simulink model "MovementCoord"  (R2016a)
settings: Solver=VariableStepAuto  SolverMode=SingleTasking  StartTime=0.0  StopTime=10.0  RelTol=1e-3
libraries: vrlib x1
settings Model: Creator=HP  LastModifiedBy=kavits
settings DebuggingCC: AlgebraicLoopMsg=none  SFUnexpectedBacktrackingDiag=error  SFNoUnconditionalDefaultTransitionDiag=error
settings GRTTargetCC: TargetLangStandard=C99 (ISO)  GeneratePreprocessorConditionals=Use local settings
settings ConfigComp: CovMetricSettings=dwe  CovHtmlReporting=off  CovSaveCumulativeToWorkspaceVar=off  CovSaveSingleToWorkspaceVar=off  CovExternalEMLEnable=on

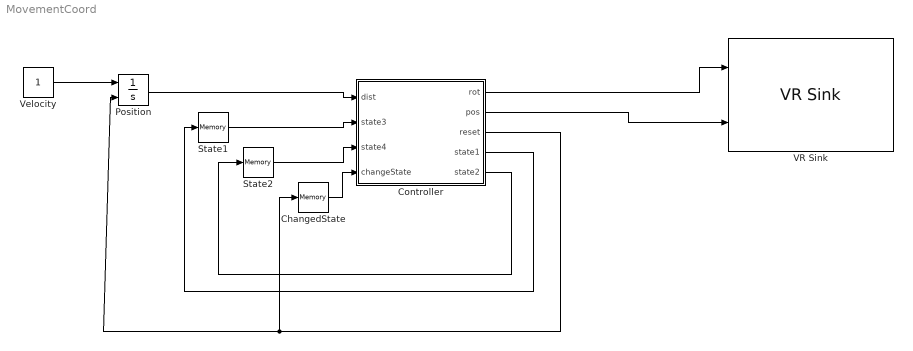
== system MovementCoord ==
  ChangedState : Memory  X0=1  InheritSampleTime=on  LinearizeMemory=on
  Controller : MATLAB Function  TreatAsAtomicUnit=on
  Position : Integrator  ExternalReset=rising
  State1 : Memory  X0=1  InheritSampleTime=on  LinearizeMemory=on
  State2 : Memory  X0=1  InheritSampleTime=on  LinearizeMemory=on
  VR Sink : vrlib/VR Sink  InstantiateOnLoad=on  SampleTime=0.0001  ViewEnable=on  RemoteChange=off  RemoteView=off  FieldsWritten=Ball.rotation.4.1.1.double#Ball.translation.3.1.1.double  WorldFileName=balls.wrl  AutoView=off  VideoDimensions=[]  AllowVariableSize=off  FigureProperties="{'Position', 'Name', 'Viewpoint', 'CameraBound', 'CameraDirection', 'CameraPosition', 'CameraUpVector', 'ZoomFactor', 'Antialiasing', 'Headlight', 'Lighting', 'NavPanel', 'Sound', 'StatusBar', 'Stereo3D', 'Stereo3DCameraOffset', 'Stereo3DHIT', 'ToolBar', 'Textures', 'Transparency', 'Triad', 'Wireframe', 'NavZones', 'NavMode', 'NavSpeed', 'CaptureFileFormat', 'CaptureFileName', 'Record2DCompressMethod', 'Record2DCompressQuality', 'Record2D', 'Record2DFileName', 'Record2DFPS'; [1.0000000000000000e+00   7.6000000000000000e+01   1.3660000000000000e+03   6.0100000000000000e+02], '', '_untitled_1', 'on', [0.0000000000000000e+00   0.0000000000000000e+00  -1.0000000000000000e+00], [0.0000000000000000e+00   0.0000000000000000e+00   0.0000000000000000e+00], [0.0000000000000000e+00   1.0000000000000000e+00   0.0000000000000000e+00], [1.0000000000000000e+00], 'on', 'on', 'on', 'halfbar', 'on', 'on', 'off', [1.0000000149011612e-01], [0.0000000000000000e+00], 'on', 'on', 'on', 'none', 'off', 'off', 'fly', 'normal', 'tif', '%f_anim_%n.tif', 'auto', [7.5000000000000000e+01], 'off', '%f_anim_%n.avi', 'auto'}"
  Velocity : Constant
  wires:
  Velocity/1 -> Position/1
  Position/1 -> Controller/1(dist)
  Controller/1(rot) -> VR Sink/1
  Controller/2(pos) -> VR Sink/2
  Controller/3(reset) -> ChangedState/1, Position/2
  Controller/5(state2) -> State2/1
  Controller/4(state1) -> State1/1
  State2/1 -> Controller/3(state4)
  State1/1 -> Controller/2(state3)
  ChangedState/1 -> Controller/4(changeState)

== matlab function MovementCoord/Controller ==
  data: rot output size=[1 4]; dist input; pos output size=[1 3]; reset output; state1 output size=1; state2 output size=1; state3 input size=1; state4 input size=1; changeState input
function [rot,pos, reset, state1, state2] = fcn(dist, state3, state4, changeState)
 
    %Variables csOut and changeState enable the simultion to know when to
    %change the starting and end positions of the ball. It is a feed/back
    %variable
    
    %nrOfEndPos = size(endPos);
    %nrOfStartPos = size(startPos);
    nrOfEndPos = 5;
    nrOfStartPos = 5;
    
    if changeState == 1
        
        %set state
        state2 = state4 + 1;
        state1 = state3;
        if state2 > nrOfEndPos
            state1 = state3 + 1;
            state2 = 1;
            if state1 > nrOfStartPos
                state1 = 1;
                state2 = 1;
            end
        end
    else
        state2 = state4;
        state1 = state3;
    end

    cameraZ = 42; %Ball needs to arrive at the given positions on the same Z as the camera
    sampleTime = 0.001;  % this parameter determines the length and the speed of the animation
                        % set outside matlabScript
    reset = 0;

    
    startInPos = 1;
    finishInPos = 1;
   
    startPos = [-24, 1.25, -20 ;-12, 1.25, -20 ; 0, 1.25, -20; 12, 1.25, -20 ; 24, 1.25, -20 ];
    endPos = [-24, 1.25, -80; -12, 1.25, -80; 0, 1.25, -80; 12, 1.25, -80; 24, 1.25, -80;];





    speed = 2 / sampleTime;
        % The bellow 3 lines control the position of the rolling ball
        % y is constant, as the ball rolls on a surface
        % the absolute value terms represent the cos and sin of the angle at which
        % the ball is rolling as seen from its starting point. (uses Pythagoras'
        % theorem)
    z = startPos(startInPos, 3) + dist * speed * ( abs(endPos(finishInPos, 3) - startPos(startInPos, 3)) / sqrt(power(startPos(startInPos, 1) - endPos(finishInPos, 1) ,2) + power(startPos(startInPos, 3) - cameraZ, 2)));
    x = startPos(startInPos, 1) + dist * speed *( (endPos(finishInPos, 1) - startPos(startInPos, 1)) / sqrt(power(startPos(startInPos, 1) - endPos(finishInPos, 1),2) + power(startPos(startInPos, 3) - cameraZ, 2)));
    y = 1.25;




    pos = [x, y, z];
    rot = [1, 0,0, dist * speed * pi/6];
    travelledZ = z;

    if travelledZ > 70 
        %reset animation
        reset = 1;

    end
    
    
    
end
